simulink model "kurs_work"  (R2022a)
settings: Solver=VariableStepAuto  StartTime=0.0  StopTime=10.0  RelTol=1e-3
values from neighbouring files (symbols this model uses):
  A = [0 1;4 3]    [untitled.m]
  B = [-3 2;1 1]    [untitled.m]
  C = [-1 0;3 1]    [untitled.m]
  D = [-4 0;0 1]    [untitled.m]
  E = [-4 2;1 0]    [untitled.m]
  F = [2 0;0 -2]    [untitled.m]
undefined symbols (not defined in the file or in its folder): A_, B_, B_f, E_, Gamma, H1, H2, Hg, K, L, L_, z_0
settings Model: Creator=Дмитрий  LastModifiedBy=Дмитрий

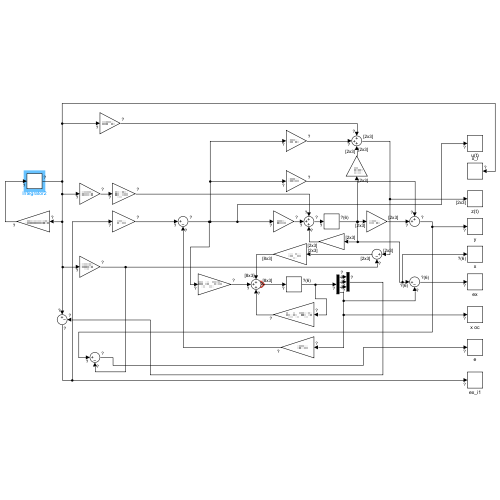
[thumbnail: Simulink's stored preview of the top-level diagram]
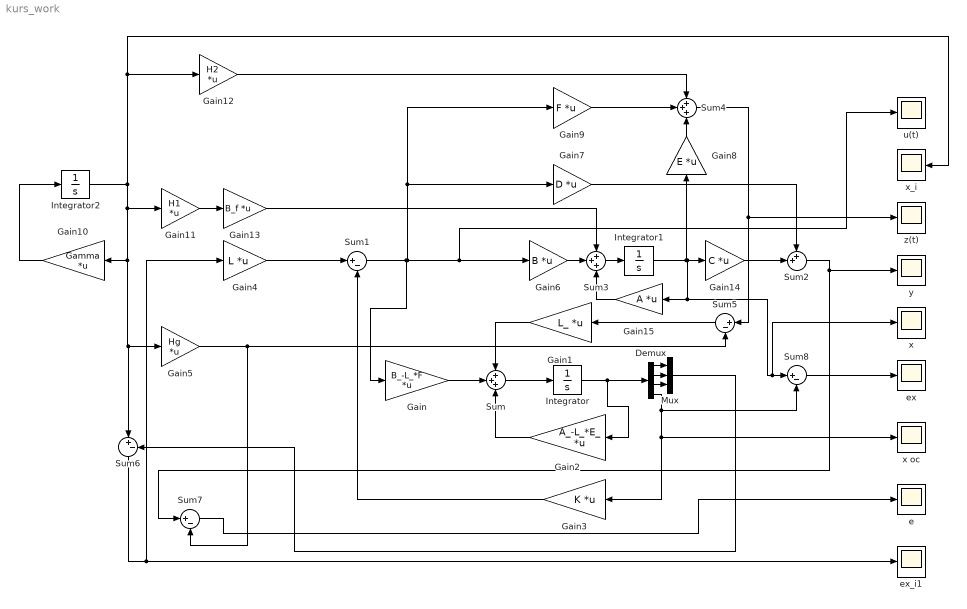
== system kurs_work ==
  Demux : Demux
  Gain : Gain  Gain=B_-L_*F  Multiplication=Matrix(K*u)
  Gain1 : Gain  Gain=L_  Multiplication=Matrix(K*u)
  Gain10 : Gain  Gain=Gamma  Multiplication=Matrix(K*u)
  Gain11 : Gain  Gain=H1  Multiplication=Matrix(K*u)
  Gain12 : Gain  Gain=H2  Multiplication=Matrix(K*u)
  Gain13 : Gain  Gain=B_f  Multiplication=Matrix(K*u)
  Gain14 : Gain  Gain=C  Multiplication=Matrix(K*u)
  Gain15 : Gain  Gain=A  Multiplication=Matrix(K*u)
  Gain2 : Gain  Gain=A_-L_*E_  Multiplication=Matrix(K*u)
  Gain3 : Gain  Gain=K  Multiplication=Matrix(K*u)
  Gain4 : Gain  Gain=L  Multiplication=Matrix(K*u)
  Gain5 : Gain  Gain=Hg  Multiplication=Matrix(K*u)
  Gain6 : Gain  Gain=B  Multiplication=Matrix(K*u)
  Gain7 : Gain  Gain=D  Multiplication=Matrix(K*u)
  Gain8 : Gain  Gain=E  Multiplication=Matrix(K*u)
  Gain9 : Gain  Gain=F  Multiplication=Matrix(K*u)
  Integrator : Integrator  InitialCondition=z_0
  Integrator1 : Integrator  InitialCondition=z_0
  Integrator2 : Integrator
  Mux : Mux  Inputs=3
  Sum : Sum  Inputs=+++
  Sum{1,5..8} (5 alike) : Sum  Inputs=|+-
  Sum2 : Sum  Inputs=++|
  Sum3 : Sum  Inputs=+++
  Sum4 : Sum  Inputs=+++
  e : Scope
  ex : Scope
  ex_i1 : Scope
  u(t) : Scope
  x : Scope
  x oc : Scope
  x_i : Scope
  y : Scope
  z(t) : Scope
  wires:
  Demux/1 -> Mux/1
  Demux/2 -> Mux/2
  Demux/3 -> Mux/3
  Gain/1 -> Sum/2
  Gain1/1 -> Sum/1
  Gain2/1 -> Sum/3
  Sum/1 -> Integrator/1
  Integrator/1 -> Gain2/1, Demux/1
  Mux/1 -> Sum6/2
  Demux/4 -> Sum8/2, Gain3/1, x oc/1
  Gain3/1 -> Sum1/2
  Gain4/1 -> Sum1/1
  Sum1/1 -> Gain/1, Gain9/1, Gain7/1, u(t)/1, Gain6/1
  Gain7/1 -> Sum2/1
  Gain6/1 -> Sum3/2
  Sum3/1 -> Integrator1/1
  Integrator1/1 -> x/1, Sum8/1, Gain15/1, Gain14/1, Gain8/1
  Gain8/1 -> Sum4/3
  Gain9/1 -> Sum4/2
  Sum5/1 -> Gain1/1
  Sum4/1 -> Sum5/1, z(t)/1
  Gain10/1 -> Integrator2/1
  Integrator2/1 -> x_i/1, Gain12/1, Sum6/1, Gain5/1, Gain10/1, Gain11/1
  Gain11/1 -> Gain13/1
  Gain13/1 -> Sum3/1
  Gain12/1 -> Sum4/1
  Gain5/1 -> Sum5/2, Sum7/2
  Sum6/1 -> Gain4/1, ex_i1/1
  Gain14/1 -> Sum2/2
  Sum2/1 -> Sum7/1, y/1
  Gain15/1 -> Sum3/3
  Sum8/1 -> ex/1
  Sum7/1 -> e/1
